simulink model "testing_model_Assignment2"  (R2022b)
settings: Solver=FixedStepAuto  StartTime=0.0  StopTime=10.0  FixedStep=1e-3  RelTol=1e-3  EnableMultiTasking=on
undefined symbols (not defined in the file): D0, D1, D10, D11, D12, D13, D2, D3, D4, D5, D6, D7, D8, D9, magnitude, PTA0, PTA1, PTA2, PTB23, PTB9, PTC16, PTC17, PTC2, PTC3, PTC4, PTD0, PTD1, PTD2, PTD3
libraries: frdmk64flib x15, dspstat3 x1
settings Model: ExtModeTrigDuration=5  Creator=clara  LastModifiedBy=pragy
settings OptimizationCC: EnhancedBackFolding=on  PassReuseOutputArgsAs=Individual arguments  ZeroExternalMemoryAtStartup=off  ZeroInternalMemoryAtStartup=off  MaxStackSize=64  OptimizeBlockOrder=speed  DifferentSizesBufferReuse=on  OptimizationCustomize=off  EfficientTunableParamExpr=on
settings DebuggingCC: ParameterTunabilityLossMsg=error
settings HardwareCC: ProdBitPerPointer=32  ProdBitPerSizeT=32  ProdBitPerPtrDiffT=32  ProdLargestAtomicInteger=Long  ProdLargestAtomicFloat=Double  ProdWordSize=32  ProdHWDeviceType=ARM Compatible->ARM Cortex
settings ModelReferenceCC: EnableRefExpFcnMdlSchedulingChecks=on
settings SFSimCC: MATLABDynamicMemAlloc=off
settings RTWCC: Description=Embedded Coder  SystemTargetFile=ert.tlc  HardwareBoard=NXP FRDM-K64F  TLCOptions="-aInlineSetEventsForThisBaseRateFcn=TLC_FALSE -aSuppressMultiTaskScheduler=TLC_FALSE  -aRateBasedStepFcn=0"  TemplateMakefile=ert_default_tmf  Toolchain=GNU Tools for ARM Embedded Processors
settings CodeAppCC: ForceParamTrailComments=on  IgnoreCustomStorageClasses=off  OperatorAnnotations=on  SimulinkDataObjDesc=on  SFDataObjDesc=on  InsertBlockDesc=on
settings ERTTargetCC: ExtModeTransport=4  ExtModeMexFile=sendToCommService

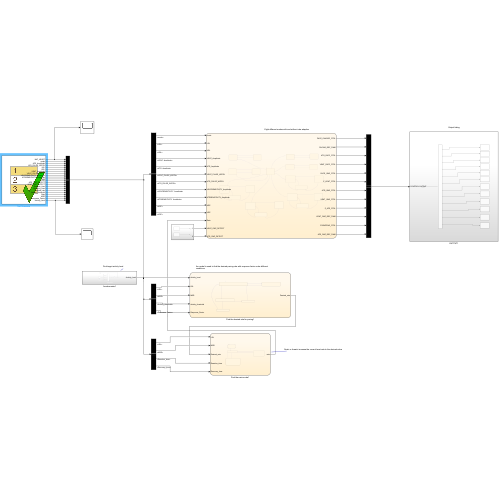
[thumbnail: Simulink's stored preview of the top-level diagram]
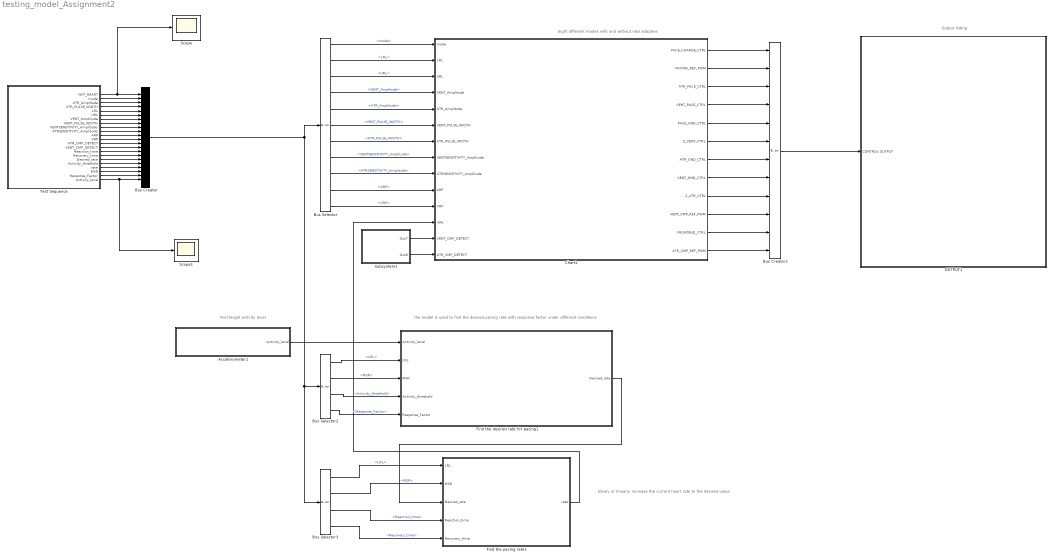
== system testing_model_Assignment2 ==
  note: Eight different modes with and without rate adaptive
  note: Slowly or linearly increase the current heart rate to the desired value
  note: Find target activity level
  note: the model is used to find the desired pacing rate with response factor under different conditions
  note: Output hiding
  Accelerometer1 : Subsystem
  Bus Creator : BusCreator  Inputs=22
  Bus Creator1 : BusCreator  Inputs=12
  Bus Selector : BusSelector  OutputSignals=mode,LRL,URL,VENT_Amplitude,ATR_Amplitude,VENT_PULSE_WIDTH,ATR_PULSE_WIDTH,VENTSENSITIVITY_Amplitude,ATRSENSITIVITY_Amplitude,ARP,VRP
  Bus Selector2 : BusSelector  OutputSignals=LRL,MSR,Activity_threshold,Response_Factor
  Bus Selector3 : BusSelector  OutputSignals=LRL,MSR,Reaction_time,Recovery_time
  Chart1 : Stateflow chart  TreatAsAtomicUnit=on
      settings: PortSchema="{\"entries\":[{\"content\":{\"sides\":[{\"content\":{\"connectorIds\":[\"In8\",\"In1\",\"In6\",\"In2\",\"In3\",\"In4\",\"In5\",\"In7\",\"In9\",\"In10\",\"In11\",\"In12\",\"In13\",\"In14\"]},\"type\":\"ConnectorPlacement.EquallySpacedRectSide\",\"uuid\":\"411cfc43-89c3-4653-9fab-0da98be593d3\"},{\"content\":{\"connectorIds\":[\"Out1\",\"Out2\",\"Out3\",\"Out4\",\"Out5\",\"Out6\",\"Out7\",\"Out8\",\"Out9\",\"Out10\",\"Out11\",\"Out12\"],\"side\":\"RIGHT\"},\"type\":\"ConnectorPlacement.EquallySpacedRectSide\",\"uuid\":\"ad1683f7-26aa-4767-b656-f3b731cb8235\"},{\"content\":{\"connectorIds\":[],\"side\":\"TOP\"},\"type\":\"ConnectorPlacement.EquallySpacedRectSide\",\"uuid\":\"fbccba07-c1cc-4c9f-8e56-0bdfb6912bb8\"}]},\"type\":\"ConnectorPlacement.EquallySpacedConnector\",\"uuid\":\"0c618a7f-9484-4de3-a6ac-3c8308721375\"}],\"packageUris\":[\"http://schema.mathworks.com/mf0/Connector/R2020b\"],\"version\":\"1.0\"}"
  Find the desired rate for pacing1 : Stateflow chart  TreatAsAtomicUnit=on
  Find the pacing rate1 : Stateflow chart  TreatAsAtomicUnit=on
  OUTPUT1 : Subsystem
  Scope : Scope
  Scope1 : Scope
  Subsystem1 : Subsystem
  Test Sequence : Test Sequence  TreatAsAtomicUnit=on
  wires:
  Bus Creator1/1 -> OUTPUT1/1(CONTROL OUTPUT)
  Chart1/11(FRONTEND_CTRL) -> Bus Creator1/11
  Chart1/12(ATR_CMP_REF_PWM) -> Bus Creator1/12
  Chart1/8(VENT_GND_CTRL) -> Bus Creator1/8
  Chart1/1(PACE_CHARGE_CTRL) -> Bus Creator1/1
  Bus Selector/6 -> Chart1/4(VENT_PULSE_WIDTH)  "<VENT_PULSE_WIDTH>"
  Chart1/10(VENT_CMP_REF_PWM) -> Bus Creator1/10
  Bus Selector2/4 -> Find the desired rate for pacing1/5(Response_Factor)  "<Response_Factor>"
  Bus Selector/8 -> Chart1/7(VENTSENSITIVITY_Amplitude)  "<VENTSENSITIVITY_Amplitude>"
  Bus Selector3/4 -> Find the pacing rate1/5(Recovery_time)  "<Recovery_time>"
  Bus Selector2/1 -> Find the desired rate for pacing1/2(LRL)  "<LRL>"
  Bus Selector3/2 -> Find the pacing rate1/2(MSR)  "<MSR>"
  Chart1/7(ATR_GND_CTRL) -> Bus Creator1/7
  Bus Selector3/3 -> Find the pacing rate1/4(Reaction_time)  "<Reaction_time>"
  Chart1/5(PACE_GND_CTRL) -> Bus Creator1/5
  Chart1/4(VENT_PACE_CTRL) -> Bus Creator1/4
  Chart1/9(Z_ATR_CTRL) -> Bus Creator1/9
  Bus Selector2/3 -> Find the desired rate for pacing1/4(Activity_threshold)  "<Activity_threshold>"
  Chart1/2(PACING_REF_PWM) -> Bus Creator1/2
  Bus Selector/11 -> Chart1/11(VRP)  "<VRP>"
  Bus Selector2/2 -> Find the desired rate for pacing1/3(MSR)  "<MSR>"
  Bus Selector3/1 -> Find the pacing rate1/1(LRL)  "<LRL>"
  Bus Selector/1 -> Chart1/8(mode)  "<mode>"
  Find the desired rate for pacing1/1(Desired_rate) -> Find the pacing rate1/3(Desired_rate)
  Chart1/6(Z_VENT_CTRL) -> Bus Creator1/6
  Bus Selector/5 -> Chart1/3(ATR_Amplitude)  "<ATR_Amplitude>"
  Chart1/3(ATR_PACE_CTRL) -> Bus Creator1/3
  Bus Selector/9 -> Chart1/9(ATRSENSITIVITY_Amplitude)  "<ATRSENSITIVITY_Amplitude>"
  Bus Selector/7 -> Chart1/5(ATR_PULSE_WIDTH)  "<ATR_PULSE_WIDTH>"
  Bus Selector/4 -> Chart1/2(VENT_Amplitude)  "<VENT_Amplitude>"
  Bus Selector/10 -> Chart1/10(ARP)  "<ARP>"
  Bus Selector/3 -> Chart1/6(URL)  "<URL>"
  Find the pacing rate1/1(rate) -> Chart1/12(rate)
  Subsystem1/2(Out8) -> Chart1/14(ATR_CMP_DETECT)
  Bus Selector/2 -> Chart1/1(LRL)  "<LRL>"
  Accelerometer1/1(Activity_level) -> Find the desired rate for pacing1/1(Activity_level)
  Subsystem1/1(Out7) -> Chart1/13(VENT_CMP_DETECT)
  Bus Creator/1 -> Bus Selector3/1, Bus Selector2/1, Bus Selector/1
  Test Sequence/1(NAT_HEART) -> Scope/1, Bus Creator/1
  Test Sequence/2(mode) -> Bus Creator/2
  Test Sequence/3(ATR_Amplitude) -> Bus Creator/3
  Test Sequence/4(ATR_PULSE_WIDTH) -> Bus Creator/4
  Test Sequence/5(LRL) -> Bus Creator/5
  Test Sequence/6(URL) -> Bus Creator/6
  Test Sequence/7(VENT_Amplitude) -> Bus Creator/7
  Test Sequence/8(VENT_PULSE_WIDTH) -> Bus Creator/8
  Test Sequence/9(VENTSENSITIVITY_Amplitude) -> Bus Creator/9
  Test Sequence/10(ATRSENSITIVITY_Amplitude) -> Bus Creator/10
  Test Sequence/11(ARP) -> Bus Creator/11
  Test Sequence/12(VRP) -> Bus Creator/12
  Test Sequence/13(ATR_CMP_DETECT) -> Bus Creator/13
  Test Sequence/14(VENT_CMP_DETECT) -> Bus Creator/14
  Test Sequence/15(Reaction_time) -> Bus Creator/15
  Test Sequence/16(Recovery_time) -> Bus Creator/16
  Test Sequence/17(Desired_rate) -> Bus Creator/17
  Test Sequence/18(Activity_threshold) -> Bus Creator/18
  Test Sequence/19(rate) -> Bus Creator/19
  Test Sequence/20(MSR) -> Bus Creator/20
  Test Sequence/22(Activity_level) -> Scope1/1, Bus Creator/22
  Test Sequence/21(Response_Factor) -> Bus Creator/21

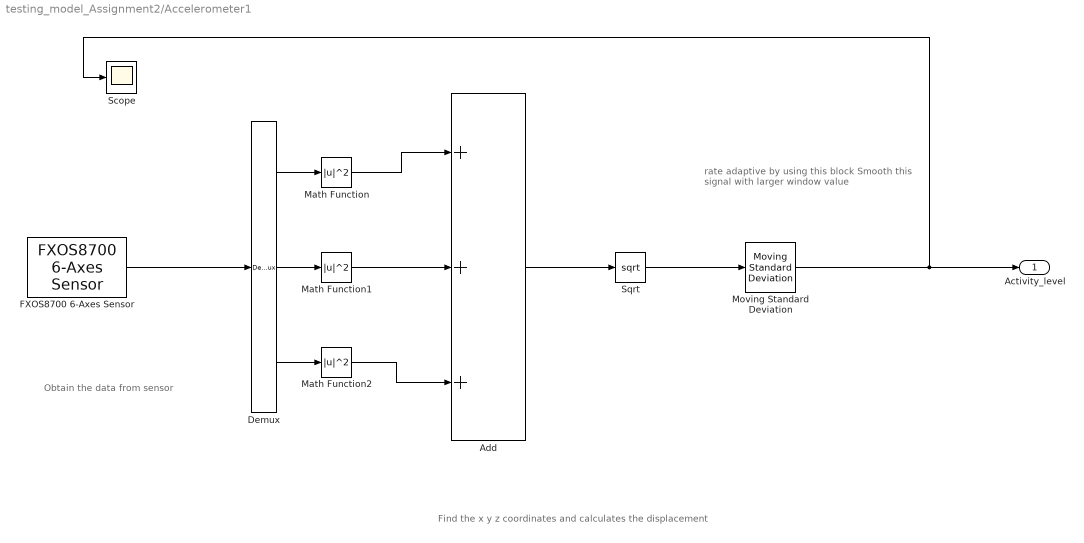
== system testing_model_Assignment2/Accelerometer1 ==
  note: Obtain the data from sensor
  note: Find the x y z coordinates and calculates the displacement
  note: rate adaptive by using this block
      | Smooth this signal with larger window value
  Add : Sum  Inputs=+++  OutDataTypeStr=double
  Demux : Demux  Outputs=3
  FXOS8700 6-Axes Sensor : frdmk64flib/FXOS8700 6-Axes Sensor  Activesensor=Accelerometer only  ODR=800Hz  HybridODR=400Hz  Accelfullrange=-4g to +4g  SampleTime=0.01
  Math Function : Math  Operator=magnitude^2  OutDataTypeStr=double
  Math Function1 : Math  Operator=magnitude^2  OutDataTypeStr=double
  Math Function2 : Math  Operator=magnitude^2  OutDataTypeStr=double
  Moving Standard Deviation : dspstat3/Moving Standard Deviation  Method=Sliding window  ForgettingFactorPort=off  SpecifyWindowLength=on  WindowLength=400  OverlapLength=399  AllowArbitraryInputLength=off  ForgettingFactor=0.9  SimulateUsing=Code generation
  Scope : Scope
  Sqrt : Sqrt  OutDataTypeStr=double
  Activity_level : Outport  OutDataTypeStr=double
  wires:
  FXOS8700 6-Axes Sensor/1 -> Demux/1
  Demux/1 -> Math Function/1
  Demux/2 -> Math Function1/1
  Demux/3 -> Math Function2/1
  Math Function/1 -> Add/1
  Math Function2/1 -> Add/3
  Math Function1/1 -> Add/2
  Add/1 -> Sqrt/1
  Sqrt/1 -> Moving Standard Deviation/1
  Moving Standard Deviation/1 -> Scope/1, Activity_level/1

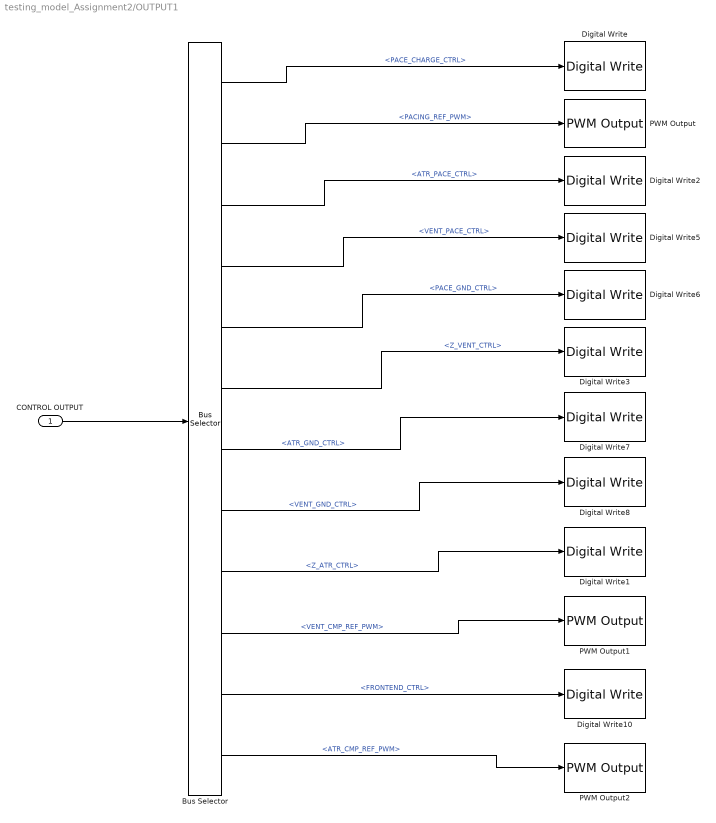
== system testing_model_Assignment2/OUTPUT1 ==
  CONTROL OUTPUT : Inport
  Bus Selector : BusSelector  OutputSignals=PACE_CHARGE_CTRL,PACING_REF_PWM,ATR_PACE_CTRL,VENT_PACE_CTRL,PACE_GND_CTRL,Z_VENT_CTRL,ATR_GND_CTRL,VENT_GND_CTRL,Z_ATR_CTRL,VENT_CMP_REF_PWM,FRONTEND_CTRL,ATR_CMP_REF_PWM
  Digital Write : frdmk64flib/Digital Write  Whichpin=PTB9 (D2)
  Digital Write1 : frdmk64flib/Digital Write  Whichpin=PTB23 (D4)
  Digital Write10 : frdmk64flib/Digital Write  Whichpin=PTD1 (D13)
  Digital Write2 : frdmk64flib/Digital Write  Whichpin=PTA0 (D8)
  Digital Write3 : frdmk64flib/Digital Write  Whichpin=PTC3 (D7)
  Digital Write5 : frdmk64flib/Digital Write  Whichpin=PTC4 (D9)
  Digital Write6 : frdmk64flib/Digital Write  Whichpin=PTD0 (D10)
  Digital Write7 : frdmk64flib/Digital Write  Whichpin=PTD2 (D11)
  Digital Write8 : frdmk64flib/Digital Write  Whichpin=PTD3 (D12)
  PWM Output : frdmk64flib/PWM Output  Whichpin=PTA2 (D5)  InitialFrequency=2000  InitialDutyCycle=0
  PWM Output1 : frdmk64flib/PWM Output  Whichpin=PTA1 (D3)  InitialFrequency=2000  InitialDutyCycle=0
  PWM Output2 : frdmk64flib/PWM Output  Whichpin=PTC2 (D6)  InitialFrequency=2000  InitialDutyCycle=0
  wires:
  CONTROL OUTPUT/1 -> Bus Selector/1
  Bus Selector/1 -> Digital Write/1  "<PACE_CHARGE_CTRL>"
  Bus Selector/2 -> PWM Output/1  "<PACING_REF_PWM>"
  Bus Selector/3 -> Digital Write2/1  "<ATR_PACE_CTRL>"
  Bus Selector/4 -> Digital Write5/1  "<VENT_PACE_CTRL>"
  Bus Selector/5 -> Digital Write6/1  "<PACE_GND_CTRL>"
  Bus Selector/6 -> Digital Write3/1  "<Z_VENT_CTRL>"
  Bus Selector/7 -> Digital Write7/1  "<ATR_GND_CTRL>"
  Bus Selector/8 -> Digital Write8/1  "<VENT_GND_CTRL>"
  Bus Selector/9 -> Digital Write1/1  "<Z_ATR_CTRL>"
  Bus Selector/10 -> PWM Output1/1  "<VENT_CMP_REF_PWM>"
  Bus Selector/11 -> Digital Write10/1  "<FRONTEND_CTRL>"
  Bus Selector/12 -> PWM Output2/1  "<ATR_CMP_REF_PWM>"

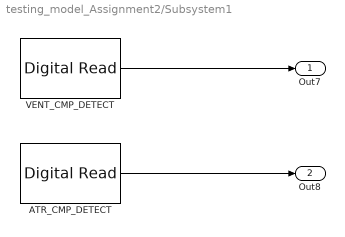
== system testing_model_Assignment2/Subsystem1 ==
  ATR_CMP_DETECT : frdmk64flib/Digital Read  Whichpin=PTC16 (D0)  SampleTime=-1
  VENT_CMP_DETECT : frdmk64flib/Digital Read  Whichpin=PTC17 (D1)  SampleTime=-1
  Out7 : Outport
  Out8 : Outport  Port=2
  wires:
  ATR_CMP_DETECT/1 -> Out8/1
  VENT_CMP_DETECT/1 -> Out7/1

== stateflow chart testing_model_Assignment2/Test Sequence ==
  state AOO
    state step_1
      mode = 1;
      ATR_Amplitude = 4;
      ATR_PULSE_WIDTH = 0.12;
      NAT_HEART = 30;
      LRL = 60;
      URL = 120;
    state step_2
      mode = 1;
      ATR_Amplitude = 4;
      ATR_PULSE_WIDTH = 0.12;
      NAT_HEART = 30;
      LRL = 60;
      URL = 120;
    (default) -> AOO.step_1
    AOO.step_1 -> AOO.step_2 : [
        | 60000/LRL - ATR_PULSE_WIDTH
        | ]
    AOO.step_2 -> AOO.step_1 : [
        | ATR_PULSE_WIDTH
        | ]
  state VOO
    state step_1
      mode = 2;
      VENT_Amplitude = 3.5;
      VENT_PULSE_WIDTH = 0.1;
      NAT_HEART = 50;
      LRL = 40;
      URL = 60;
    state step_2
      mode = 2;
      VENT_Amplitude = 3.5;
      VENT_PULSE_WIDTH = 0.1;
      NAT_HEART = 50;
      LRL = 40;
      URL = 60;
    (default) -> VOO.step_1
    VOO.step_1 -> VOO.step_2 : [
        | 60000/LRL - VENT_PULSE_WIDTH
        | ]
    VOO.step_2 -> VOO.step_1 : [
        | VENT_PULSE_WIDTH
        | ]
  state AAI
    state Charging
      mode = 3;
      ATR_Amplitude = 4.5;
      ATR_PULSE_WIDTH = 1.5;
      ATRSENSITIVITY_Amplitude = 0.5;
      ARP = 150;
      NAT_HEART = 40;
      LRL = 60;
      URL = 120;
      state No_natural_heartbeat
        ATR_CMP_DETECT = 0;
      state Natrural_hearbeat
        ATR_CMP_DETECT = 1;
      (default) -> AAI.Charging.No_natural_heartbeat
      AAI.Charging.No_natural_heartbeat -> AAI.Charging.Natrural_hearbeat : [
          | 60000/LRL - ATR_PULSE_WIDTH - double(ARP)
          | ]
      AAI.Charging.Natrural_hearbeat -> AAI.Charging.No_natural_heartbeat : [
          | ARP
          | ]
    state Pacing
      mode = 3;
      ATR_Amplitude = 4.5;
      ATR_PULSE_WIDTH = 1.5;
      ATRSENSITIVITY_Amplitude = 0.5;
      ARP = 150;
      NAT_HEART = 40;
      LRL = 60;
      URL = 120;
    state Refractory
      mode = 3;
      ATR_Amplitude = 4.5;
      ATR_PULSE_WIDTH = 1.5;
      ATRSENSITIVITY_Amplitude = 0.5;
      ARP = 150;
      NAT_HEART = 40;
      LRL = 60;
      URL = 120;
    (default) -> AAI.Charging
    (junction 108) -> AAI.Charging
    AAI.Pacing -> AAI.Refractory : [
        | ARP
        | ]
    AAI.Refractory -> (junction 110) : [
        | ARP
        | ]
    (junction 110) -> (junction 108)
  state VVI
    state Charging
      mode = 4;
      VENT_Amplitude = 4;
      VENT_PULSE_WIDTH = 1;
      VENTSENSITIVITY_Amplitude = 0.75;
      VRP = 400;
      NAT_HEART = 80;
      LRL = 70;
      URL = 160;
      state No_natural_heartbeat
        VENT_CMP_DETECT = 0;
      state Natrural_hearbeat
        VENT_CMP_DETECT = 1;
      (default) -> VVI.Charging.No_natural_heartbeat
      VVI.Charging.No_natural_heartbeat -> VVI.Charging.Natrural_hearbeat : [
          | 60000/LRL - VENT_PULSE_WIDTH - double(VRP)
          | ]
      VVI.Charging.Natrural_hearbeat -> VVI.Charging.No_natural_heartbeat : [
          | VRP
          | ]
    state Pacing
      mode = 4;
      VENT_Amplitude = 4;
      VENT_PULSE_WIDTH = 1;
      VENTSENSITIVITY_Amplitude = 0.75;
      VRP = 400;
      NAT_HEART = 80;
      LRL = 70;
      URL = 160;
    state Refractory
      mode = 4;
      VENT_Amplitude = 4;
      VENT_PULSE_WIDTH = 1;
      VENTSENSITIVITY_Amplitude = 0.75;
      VRP = 400;
      NAT_HEART = 80;
      LRL = 70;
      URL = 160;
    (default) -> VVI.Charging
    (junction 141) -> VVI.Charging
    VVI.Pacing -> VVI.Refractory : [
        | VRP
        | ]
    VVI.Refractory -> (junction 143) : [
        | VRP
        | ]
    (junction 143) -> (junction 141)
  state AOOR
    state step_1
      mode = 5;
      Desired_rate = 70;
      ATR_Amplitude = 3.5;
      ATR_PULSE_WIDTH = 0.3;
      NAT_HEART = 30;
      Activity_threshold = 1;
      Response_Factor = 8;
      Reaction_time = 30;
      Recovery_time = 8;
      LRL = 75;
      URL = 165;
      MSR = 65;
      state CONST_ACT_LEVEL
        Activity_level = 5;
      state Changing_Activity
        Activity_level = 5+30*sin(et*2*pi/30)
      (default) -> AOOR.step_1.CONST_ACT_LEVEL
      AOOR.step_1.CONST_ACT_LEVEL -> AOOR.step_1.Changing_Activity : [
          | et >10
          | ]
      AOOR.step_1.Changing_Activity -> AOOR.step_1.CONST_ACT_LEVEL : [
          | Activity_level < 5
          | ]
    state step_2
      mode = 5;
      Desired_rate = 70;
      ATR_Amplitude = 3.5;
      ATR_PULSE_WIDTH = 0.3;
      NAT_HEART = 30;
      Activity_threshold = 1;
      Response_Factor = 8;
      Reaction_time = 30;
      Recovery_time = 8;
      LRL = 75;
      URL = 165;
      MSR = 65;
    (default) -> AOOR.step_1
    AOOR.step_2 -> AOOR.step_1 : [
        | ATR_PULSE_WIDTH
        | ]
    AOOR.step_1 -> AOOR.step_2 : [
        | 60000/rate - ATR_PULSE_WIDTH
        | ]
  state VOOR
    state step_1
      mode = 6;
      Desired_rate = 60;
      VENT_Amplitude = 3.8;
      VENT_PULSE_WIDTH = 1.7;
      NAT_HEART = 140;
      Activity_threshold = 7;
      Response_Factor = 15;
      Reaction_time = 38;
      Recovery_time = 12;
      LRL = 40;
      URL = 100;
      MSR = 170;
      state CONST_ACT_LEVEL
        Activity_level = 5;
      state Changing_Activity
        Activity_level = 5+30*sin(et*2*pi/30)
      (default) -> VOOR.step_1.CONST_ACT_LEVEL
      VOOR.step_1.CONST_ACT_LEVEL -> VOOR.step_1.Changing_Activity : [
          | et >10
          | ]
      VOOR.step_1.Changing_Activity -> VOOR.step_1.CONST_ACT_LEVEL : [
          | Activity_level < 5
          | ]
    state step_2
      mode = 6;
      Desired_rate = 60;
      VENT_Amplitude = 3.8;
      VENT_PULSE_WIDTH = 1.7;
      NAT_HEART = 140;
      Activity_threshold = 7;
      Response_Factor = 15;
      Reaction_time = 38;
      Recovery_time = 12;
      LRL = 40;
      URL = 100;
      MSR = 170;
    (default) -> VOOR.step_1
    VOOR.step_1 -> VOOR.step_2 : [
        | 60000/rate - VENT_PULSE_WIDTH
        | ]
    VOOR.step_2 -> VOOR.step_1 : [
        | VENT_PULSE_WIDTH
        | ]
  state AAIR
    state step_1
      mode = 7;
      Desired_rate = 100;
      ATR_Amplitude = 3.6;
      ATR_PULSE_WIDTH = 1.8;
      NAT_HEART = 5;
      Activity_threshold = 4;
      Response_Factor = 12;
      Reaction_time = 10;
      Recovery_time = 3;
      ARP = 150;
      ATRSENSITIVITY_Amplitude = 1.5;
      LRL = 60;
      URL = 120;
      MSR = 150;
      ATR_CMP_DETECT = 0;
      state CONST_ACT_LEVEL
        Activity_level = 5;
      state Changing_Activity
        Activity_level = 5+30*sin(et*2*pi/30)
      (default) -> AAIR.step_1.CONST_ACT_LEVEL
      AAIR.step_1.CONST_ACT_LEVEL -> AAIR.step_1.Changing_Activity : [
          | et >10
          | ]
      AAIR.step_1.Changing_Activity -> AAIR.step_1.CONST_ACT_LEVEL : [
          | Activity_level < 5
          | ]
    state step_2
    (default) -> AAIR.step_1
    AAIR.step_1 -> AAIR.step_2 : [
        | 60000/rate - ATR_PULSE_WIDTH
        | ]
  state VVIR
    state step_1
      mode = 8;
      Desired_rate = 65;
      VENT_Amplitude = 5;
      VENT_PULSE_WIDTH = 0.5;
      NAT_HEART = 65;
      Activity_threshold = 7;
      Response_Factor = 10;
      Reaction_time = 30;
      Recovery_time = 5;
      VRP = 300;
      VENTSENSITIVITY_Amplitude = 2;
      LRL = 50;
      URL = 110;
      MSR = 80;
      VENT_CMP_DETECT = 0;
      state CONST_ACT_LEVEL
        Activity_level = 3;
      state Changing_Activity
        Activity_level = 3+30*sin(et*2*pi/30)
      (default) -> VVIR.step_1.CONST_ACT_LEVEL
      VVIR.step_1.CONST_ACT_LEVEL -> VVIR.step_1.Changing_Activity : [
          | et >10
          | ]
      VVIR.step_1.Changing_Activity -> VVIR.step_1.CONST_ACT_LEVEL : [
          | Activity_level < 3
          | ]
    state step_2
    (default) -> VVIR.step_1
    VVIR.step_1 -> VVIR.step_2 : [
        | 60000/rate - VENT_PULSE_WIDTH
        | ]
  (default) -> AOO [order 1] : [Active_Scenario_Index == 1]
  (default) -> VOO [order 2] : [Active_Scenario_Index == 2]
  (default) -> AAI [order 3] : [Active_Scenario_Index == 3]
  (default) -> VVI [order 4] : [Active_Scenario_Index == 4]
  (default) -> AOOR [order 5] : [Active_Scenario_Index == 5]
  (default) -> VOOR [order 6] : [Active_Scenario_Index == 6]
  (default) -> AAIR [order 7] : [Active_Scenario_Index == 7]
  (default) -> VVIR [order 8] : {assert(Active_Scenario_Index == 8,'The value of Scenario Parameter ''Active_Scenario_Index'' is not valid. Use the index of the scenario to specify it.')}
  data: NAT_HEART output; Active_Scenario_Index parameter =1; mode output; ATR_Amplitude output; ATR_PULSE_WIDTH output; LRL output; URL output; VENT_Amplitude output; VENT_PULSE_WIDTH output; VENTSENSITIVITY_Amplitude output; ATRSENSITIVITY_Amplitude output; ARP output; VRP output; ATR_CMP_DETECT output; VENT_CMP_DETECT output; Reaction_time output; Recovery_time output; Desired_rate output; Activity_threshold output; rate output; MSR output; Response_Factor output; Activity_level output

== stateflow chart testing_model_Assignment2/Chart1 ==
  note: Pace ready
  state Pacing_AOO
    entry:
    PACE_CHARGE_CTRL = false;
    PACE_GND_CTRL = true;
    ATR_PACE_CTRL = true;
    ATR_GND_CTRL = false;
    %
  note: Pace ready
  state AOO
    entry:
    % charge condition for C22
    ATR_PACE_CTRL = false;
    PACE_CHARGE_CTRL = true;
    % discharge condition for C21;
    ATR_GND_CTRL = true;
    PACE_GND_CTRL = true;
    %
    PACING_REF_PWM = 20*ATR_Amplitude;
  state AOOR
    entry:
    % charge condition for C22
    ATR_PACE_CTRL = false;
    PACE_CHARGE_CTRL = true;
    % discharge condition for C21;
    ATR_GND_CTRL = true;
    PACE_GND_CTRL = true;
    %
    PACING_REF_PWM = 20*ATR_Amplitude;
  state Pacing_AOOR
    entry:
    PACE_CHARGE_CTRL = false;
    PACE_GND_CTRL = true;
    ATR_PACE_CTRL = true;
    ATR_GND_CTRL = false;
    %
  note: Recharge ready
  note: Recharge ready
  note: Charge C22 and discharge blocking capacitor
  note: Discharge C22 into atrium (charge C21)
  note: Pace ready
  state VOO
    entry:
    % charge condition for C22
    VENT_PACE_CTRL = false;
    PACE_CHARGE_CTRL = true;
    % discharge condition for C21;
    VENT_GND_CTRL = true;
    PACE_GND_CTRL = true;
    %
    PACING_REF_PWM = 20*VENT_Amplitude;
  state Pacing_VOO
    entry:
    PACE_CHARGE_CTRL = false;
    PACE_GND_CTRL = true;
    VENT_GND_CTRL = false;
    VENT_PACE_CTRL = true;
    %
  note: Initial conditions
  state MAIN
    entry:
    VENT_GND_CTRL=false;
    Z_ATR_CTRL = false;
    Z_VENT_CTRL = false;
    FRONTEND_CTRL=false;
    PACE_CHARGE_CTRL = false;
    VENT_PACE_CTRL = false;
    ATR_PACE_CTRL = false;
    PACE_GND_CTRL=false;
    ATR_GND_CTRL=false;
  note: Pace ready
  note: Recharge ready
  state VOOR
    entry:
    % charge condition for C22
    VENT_PACE_CTRL = false;
    PACE_CHARGE_CTRL = true;
    % discharge condition for C21;
    VENT_GND_CTRL = true;
    PACE_GND_CTRL = true;
    %
    PACING_REF_PWM = 20*VENT_Amplitude;
  state Pacing_VOOR
    entry:
    PACE_CHARGE_CTRL = false;
    PACE_GND_CTRL = true;
    VENT_GND_CTRL = false;
    VENT_PACE_CTRL = true;
    %
  note: Charge C22 and discharge blocking capacitor
  note: Discharge C22 into ventrical (charge C21)
  note: Begin sensing, charge C22 and discharge
      | blocking capacitor
  note: Discharge C22 into atrium (charge C21)
  note: If no signal is sensed
  state AAI
    entry:
    % begin sensing
    FRONTEND_CTRL = true;
    % charge condition for C22
    ATR_PACE_CTRL = false;
    PACE_CHARGE_CTRL = true;
    % discharge condition for C21;
    ATR_GND_CTRL = true;
    PACE_GND_CTRL = true;
    %
    PACING_REF_PWM = 20*ATR_Amplitude;
    ATR_CMP_REF_PWM = 20*ATRSENSITIVITY_Amplitude;
  state Pacing_AAI1
    entry:
    PACE_CHARGE_CTRL = false;
    PACE_GND_CTRL = true;
    ATR_PACE_CTRL = true;
    ATR_GND_CTRL = false;
    %
    PACING_REF_PWM = 20*ATR_Amplitude;
  note: If signal is sensed
  note: If no signal is sensed
  state AAI_REFRACTORY
    entry:
    FRONTEND_CTRL = false;
    ATR_PACE_CTRL = false;
    ATR_GND_CTRL = true;
    PACING_REF_PWM = 20*ATR_Amplitude;
    PACE_CHARGE_CTRL = false;
    PACE_GND_CTRL = true;
  state Pacing_AAIR
    entry:
    PACE_CHARGE_CTRL = false;
    PACE_GND_CTRL = true;
    ATR_PACE_CTRL = true;
    ATR_GND_CTRL = false;
    %
    PACING_REF_PWM = 20*ATR_Amplitude;
  state AAIR
    entry:
    % begin sensing
    FRONTEND_CTRL = true;
    % charge condition for C22
    ATR_PACE_CTRL = false;
    PACE_CHARGE_CTRL = true;
    % discharge condition for C21;
    ATR_GND_CTRL = true;
    PACE_GND_CTRL = true;
    %
    PACING_REF_PWM = 20*ATR_Amplitude;
    ATR_CMP_REF_PWM = 20*ATRSENSITIVITY_Amplitude;
  note: If signal is sensed
  note: Follows events during which senses
      | in the atrium are ignored
  note: If signal is sensed
  note: Begin sensing, charge C22 and discharge
      | blocking capacitor
  note: Discharge C22 into ventrical (charge C21)
  note: If no signal is sensed
  state Pacing_VVI
    entry:
    PACE_CHARGE_CTRL = false;
    PACE_GND_CTRL = true;
    VENT_GND_CTRL = false;
    VENT_PACE_CTRL = true;
    %
    PACING_REF_PWM = 20*VENT_Amplitude;
  state VVI
    entry:
    % begin sensing
    FRONTEND_CTRL = true;
    % charge condition for C22
    VENT_PACE_CTRL = false;
    PACE_CHARGE_CTRL = true;
    % discharge condition for C21;
    VENT_GND_CTRL = true;
    PACE_GND_CTRL = true;
    %
    PACING_REF_PWM = 20*VENT_Amplitude;
    VENT_CMP_REF_PWM = 20*VENTSENSITIVITY_Amplitude;
  state AAIR_REFRACTORY
    entry:
    FRONTEND_CTRL = false;
    ATR_PACE_CTRL = false;
    ATR_GND_CTRL = true;
    PACING_REF_PWM = 20*ATR_Amplitude;
    PACE_CHARGE_CTRL = false;
    PACE_GND_CTRL = true;
  note: If signal is sensed
  note: If signal is sensed
  note: Follows events during which senses
      | in the atrium are ignored
  note: If no signal is sensed
  state Pacing_VVIR
    entry:
    PACE_CHARGE_CTRL = false;
    PACE_GND_CTRL = true;
    VENT_GND_CTRL = false;
    VENT_PACE_CTRL = true;
    %
    PACING_REF_PWM = 20*VENT_Amplitude;
  state VVIR
    entry:
    % begin sensing
    FRONTEND_CTRL = true;
    % charge condition for C22
    VENT_PACE_CTRL = false;
    PACE_CHARGE_CTRL = true;
    % discharge condition for C21;
    VENT_GND_CTRL = true;
    PACE_GND_CTRL = true;
    %
    PACING_REF_PWM = 20*VENT_Amplitude;
    VENT_CMP_REF_PWM = 20*VENTSENSITIVITY_Amplitude;
  state VVI_REFRACTORY
    entry:
    FRONTEND_CTRL = false;
    VENT_GND_CTRL = true;
    PACING_REF_PWM = 20*VENT_Amplitude;
    PACE_CHARGE_CTRL = false;
    PACE_GND_CTRL = true;
  note: If signal is sensed
  note: If signal is sensed
  note: Follows events during which senses
      | in the ventrical are ignored
  state VVIR_REFRACTORY
    entry:
    FRONTEND_CTRL = false;
    VENT_GND_CTRL = true;
    PACING_REF_PWM = 20*VENT_Amplitude;
    PACE_CHARGE_CTRL = false;
    PACE_GND_CTRL = true;
  note: If signal is sensed
  AOO -> Pacing_AOO : after((60000/LRL - ATR_PULSE_WIDTH),msec)
  AOOR -> Pacing_AOOR : [after(60000/rate - ATR_PULSE_WIDTH,msec)]
  MAIN -> AOO [order 4] : [mode == 1]
  Pacing_AOO -> AOO : [after(ATR_PULSE_WIDTH,msec)]
  Pacing_AOOR -> AOOR : [after(ATR_PULSE_WIDTH,msec)]
  MAIN -> AOOR [order 5] : [mode == 5]
  VOO -> Pacing_VOO : [after(60000/LRL - VENT_PULSE_WIDTH,msec)]
  MAIN -> VOO [order 1] : [mode == 2]
  (default) -> MAIN
  Pacing_VOO -> VOO : [after(VENT_PULSE_WIDTH,msec)]
  VOOR -> Pacing_VOOR : [after(60000/rate - VENT_PULSE_WIDTH,msec)]
  Pacing_VOOR -> VOOR : [after(VENT_PULSE_WIDTH,msec)]
  MAIN -> AAI [order 3] : [mode == 3]
  MAIN -> VOOR [order 6] : [mode == 6]
  MAIN -> AAIR [order 7] : [mode == 7]
  MAIN -> VVIR [order 8] : [mode == 8]
  MAIN -> VVI [order 2] : [mode == 4]
  AAI -> Pacing_AAI1 [order 1] : [(ATR_CMP_DETECT==false) &&after(60000/LRL - ATR_PULSE_WIDTH-double(ARP),msec)]
  AAI -> AAI_REFRACTORY [order 2] : [ATR_CMP_DETECT == true]
  AAI_REFRACTORY -> AAI : [after(ARP,msec)]
  Pacing_AAI1 -> AAI_REFRACTORY : [ATR_CMP_DETECT == true]
  AAIR -> Pacing_AAIR [order 1] : [(ATR_CMP_DETECT==false) &&after(60000/rate - ATR_PULSE_WIDTH - double(ARP),msec)]
  AAIR -> AAIR_REFRACTORY [order 2] : [ATR_CMP_DETECT == true]
  Pacing_AAIR -> AAIR_REFRACTORY : [ATR_CMP_DETECT == true]
  AAIR_REFRACTORY -> AAIR : [after(ARP,msec)]
  VVI -> Pacing_VVI [order 1] : [(VENT_CMP_DETECT==false) &&after(60000/LRL - VENT_PULSE_WIDTH-double(VRP),msec)]
  VVI -> VVI_REFRACTORY [order 2] : [VENT_CMP_DETECT == true]
  Pacing_VVI -> VVI_REFRACTORY : [VENT_CMP_DETECT == true]
  VVI_REFRACTORY -> VVI : [after(VRP,msec)]
  VVIR -> Pacing_VVIR [order 1] : [(VENT_CMP_DETECT==false) &&after(60000/rate - VENT_PULSE_WIDTH-double(VRP),msec)]
  VVIR -> VVIR_REFRACTORY [order 2] : [VENT_CMP_DETECT == true]
  Pacing_VVIR -> VVIR_REFRACTORY : [VENT_CMP_DETECT == true]
  VVIR_REFRACTORY -> VVIR : [after(VRP,msec)]
  data: LRL input; VENT_Amplitude input; ATR_Amplitude input; VENT_PULSE_WIDTH input; ATR_PULSE_WIDTH input; URL input; VENTSENSITIVITY_Amplitude input; PACE_CHARGE_CTRL output; PACING_REF_PWM output; ATR_PACE_CTRL output; VENT_PACE_CTRL output; PACE_GND_CTRL output; Z_VENT_CTRL output; ATR_GND_CTRL output; VENT_GND_CTRL output; Z_ATR_CTRL output; VENT_CMP_REF_PWM output; FRONTEND_CTRL output; mode input; ATR_CMP_REF_PWM output; ATRSENSITIVITY_Amplitude input; ARP input; VRP input; rate input; VENT_CMP_DETECT input; ATR_CMP_DETECT input

== stateflow chart testing_model_Assignment2/Find the desired rate for pacing1 ==
  note: Two conditions for the comparsion
  note: If our detected level is lower than or equal to the threshold
      | The desired will not increase, it will stay at LRL
  state Desired_rate_output_3
    entry:
    Desired_rate = LRL;
  state Check
    % check how the desired rate is going to change depends on activity level
  note: Loop back to the initial state and keep checking
  note: We find a higher rate when we have a larger value than the threshold
  note: Make sure the desired rate will not larger than MSR
  state Linear_increase
    entry:
    temp_rate = LRL + Response_Factor*(Activity_level-double(Activity_threshold));
  state Desired_rate_output_2
    entry:
    Desired_rate = MSR;
  state Desired_rate_output_1
    entry:
    Desired_rate = temp_rate;
  (default) -> Check
  Check -> Desired_rate_output_3 [order 2] : [Activity_level <= Activity_threshold]
  Desired_rate_output_1 -> Check : after(300,msec)
  Desired_rate_output_3 -> Check : after(300,msec)
  Check -> Linear_increase [order 1] : [Activity_level > Activity_threshold]
  Desired_rate_output_2 -> Check : after(300,msec)
  Linear_increase -> Desired_rate_output_2 [order 2] : [temp_rate >= MSR]
  Linear_increase -> Desired_rate_output_1 [order 1] : [temp_rate < MSR]
  data: Activity_level input double; LRL input; MSR input; Activity_threshold input single; Response_Factor input; Desired_rate output; temp_rate local

== stateflow chart testing_model_Assignment2/Find the pacing rate1 ==
  state Initial_state
    rate = LRL;
  note: Firstly define the rate to LRL
  note: If the rate is larger than our desired rate, it decreases
  note: Different increments when facing various conditions
  state Steps
    entry:
    addition = (MSR-LRL)/double(Reaction_time);
    substruction = (MSR-LRL)/double(Recovery_time);
  state Decreasing
    % using linear function to decrease
    entry:
    if(rate < MSR)
    rate = rate  - substruction;
    elseif(rate <= LRL)
    rate = LRL;
    end
  note: The rate can not be smaller than LRL
  note: Keep checking for every 300 ms
  note: Do the addition if we have a higher desired rate
  state Increasing
    % using linear function to increase
    entry:
    if(rate < MSR && rate < Desired_rate)
    rate = rate + addition;
    elseif(rate == Desired_rate)
    rate = Desired_rate;
    elseif(rate >= MSR)
    rate = MSR;
    end
  note: The rate should not exceed MSR
  (default) -> Initial_state
  Initial_state -> Steps
  Steps -> Decreasing [order 1] : after(300,msec)[rate > Desired_rate]
  Decreasing -> Steps : after(300,msec)
  Steps -> Increasing [order 2] : after(300,msec)
  Increasing -> Steps : after(300,msec)
  data: LRL input; MSR input; Desired_rate input; Reaction_time input uint16; Recovery_time input uint16; rate output; addition local; substruction local
